simulink model "exampleGround_Source_Heat_Exchanger"  (Simulink 7.6)
settings: Solver=ode45  StartTime=0.0  StopTime=1*24*3600  RelTol=1e-4  AbsTol=1e-5
settings Model: Creator=drhf  LastModifiedBy=awohlfei
settings CodeAppCC: CustomSymbolStrType=$N$R$M_T

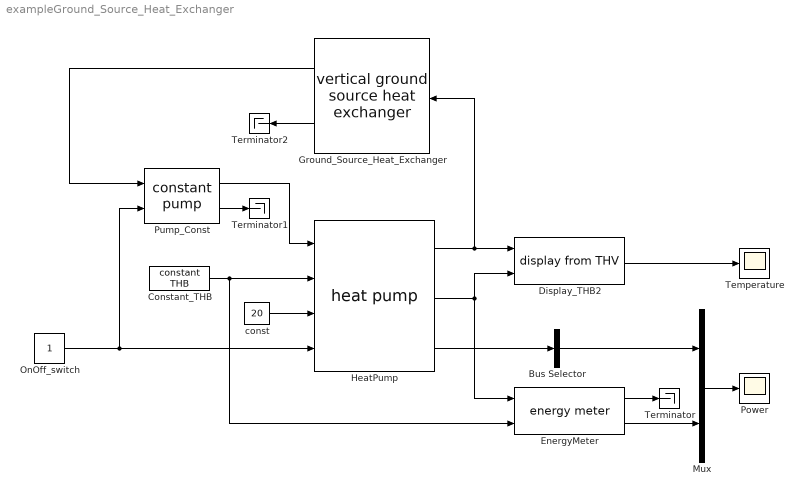
== system exampleGround_Source_Heat_Exchanger ==
  Bus Selector : BusSelector  OutputSignals=Pelec,Qdot_cold,Qdot_hot  OutputAsBus=on
  Constant_THB : Reference  SystemSampleTime=-1  t=40  mdot=900/3600  p=1e5  mID=No Pressure Drop  fluid=water  mix=0  dia=0.02  hgt=0
  Display_THB2 : Reference  SystemSampleTime=-1  t=on  m=off  p=off  id=off  mix=off  d=off
  EnergyMeter : Reference  SystemSampleTime=-1
  Ground_Source_Heat_Exchanger : Reference  SystemSampleTime=-1  Jahresmitteltemp_C=12  TGrad=0.025  lambdaErde=2.0  cpErde=800  rhoErde=2500  lambdaFill=1.0  cpFill=1000  rhoFill=2000  Sondelaenge=100  B=10  Sondendurchmesser=0.032  Bohrdurchmesser=0.18  sondenfall=1 probe  np=1  DimAxi=10  DimRad=10  Gitterfaktor=2.5
  HeatPump : Reference  SystemSampleTime=-1  Tcin=[-5 15]  Thout=[35 45 55 60]  Qdotc=[14000 12500 10000 9200;26900 24000 21700 20000]  Qdoth=[18000 17200 16500 16000;31500 29500 27800 27000]  Pel=[4400 5500 7000 7500;4600 6000 7000 7500]  caph=80000  capc=50000  UA=7  linc=10  quac=10  linh=10  quah=10
  Mux : Mux  Inputs=2
  OnOff_switch : Constant
      settings: OpenFcn=set_param(gcb,'value',num2str(1-str2num(get_param(gcb,'value'))))
  Power : Scope
      settings: TickLabels=on  YMin=-20000  YMax=20000
  Pump_Const : Reference  SystemSampleTime=-1  mdotmax=3000/3600  dia=0.0157  power=30  p0=3e5  fluid_id=water  mix=0  UA=0  mcp=0  tamb=20
  Temperature : Scope
      settings: TickLabels=on  YMin=-15  YMax=55
  Terminator : Terminator
  Terminator1 : Terminator
  Terminator2 : Terminator
  const : Constant  Value=20
  wires:
  OnOff_switch/1 -> HeatPump/4, Pump_Const/2
  Display_THB2/1 -> Temperature/1
  Mux/1 -> Power/1
  EnergyMeter/1 -> Terminator/1
  EnergyMeter/2 -> Mux/2
  Bus Selector/1 -> Mux/1
  HeatPump/3 -> Bus Selector/1
  HeatPump/1 -> Display_THB2/1, Ground_Source_Heat_Exchanger/1
  HeatPump/2 -> Display_THB2/2, EnergyMeter/1
  const/1 -> HeatPump/3
  Constant_THB/1 -> HeatPump/2, EnergyMeter/2
  Pump_Const/1 -> HeatPump/1
  Pump_Const/2 -> Terminator1/1
  Ground_Source_Heat_Exchanger/2 -> Terminator2/1
  Ground_Source_Heat_Exchanger/1 -> Pump_Const/1
